simulink model "simgoid_terry"  (R2020b)
settings: Solver=VariableStepAuto  StartTime=0.0  StopTime=200  RelTol=1e-3
values from neighbouring files (symbols this model uses):
  A_2 = zeros(3)    [Trial_Script.m]
  B_2 = I_inv    [Trial_Script.m]
  C_2 = eye(3)    [Trial_Script.m]
  D_2 = zeros(3)    [Trial_Script.m]
libraries: mpclib x1, fuzblock x1, cstblocks x1
settings Model: Creator=Jonathan van Zyl  LastModifiedBy=Jonathan van Zyl

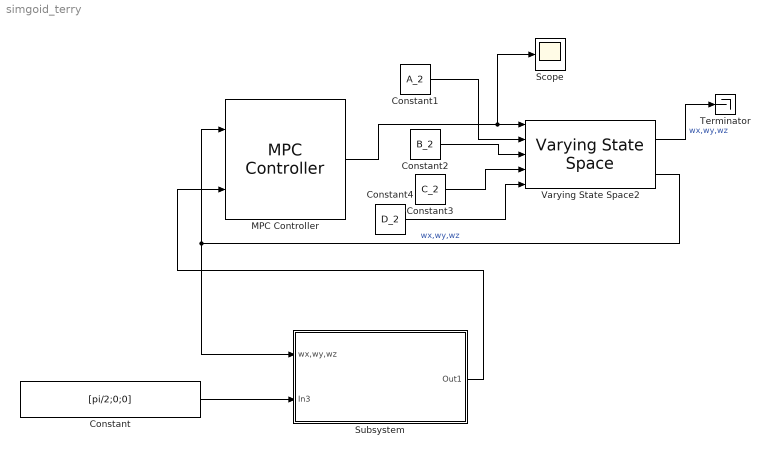
== system simgoid_terry ==
  Constant : Constant  Value=[pi/2;0;0]
  Constant1 : Constant  Value=A_2
  Constant2 : Constant  Value=B_2
  Constant3 : Constant  Value=C_2
  Constant4 : Constant  Value=D_2
  MPC Controller : mpclib/MPC Controller  SCDEnableBlockLinearizationSpecification=on  mpcobj=mpc1  is_multiple=0  enable_value=0  return_u0=off  updateMPCinCallerWorkspace=on  md_inport=off  mv_inport=off  uref_inport=off  return_cost=off  return_mvseq=off  return_qpstatus=off  return_xseq=off  return_state=off  return_ovseq=off  state_inport=off  umin_inport=off  umax_inport=off  ymin_inport=off  ymax_inport=off  cc_inport=off  ywt_inport=off  uwt_inport=off  duwt_inport=off  rhoeps_inport=off  pm_inport=off  MaximumP=10  HorizonChoice=FixedHorizon  n_ts=0.1  n_p=10  n_mv=3  n_md=0  n_ud=0  n_mo=3  n_uo=0  BlockDataType=double  SampleTimeInherited=off  switch_inport=off
  Scope : Scope
  Subsystem : Subsystem
  Terminator : Terminator
  Varying State Space2 : cstblocks/Linear Parameter Varying/Varying State Space  x0=0  xNames=''  OutputX=on  OutputDX=off
  wires:
  Constant3/1 -> Varying State Space2/4
  MPC Controller/1 -> Varying State Space2/1, Scope/1
  Constant2/1 -> Varying State Space2/3
  Varying State Space2/1 -> Terminator/1  "wx,wy,wz"
  Constant4/1 -> Varying State Space2/5
  Varying State Space2/2 -> MPC Controller/1, Subsystem/1(wx,wy,wz)  "wx,wy,wz"
  Constant1/1 -> Varying State Space2/2
  Constant/1 -> Subsystem/2(In3)
  Subsystem/1(Out1) -> MPC Controller/2

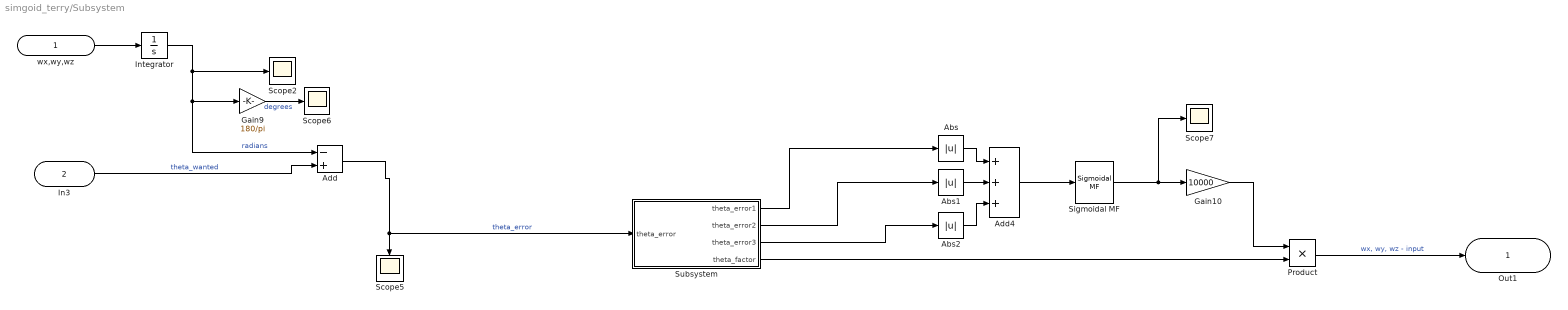
== system simgoid_terry/Subsystem ==
  wx,wy,wz : Inport
  In3 : Inport  Port=2
  Abs : Abs
  Abs1 : Abs
  Abs2 : Abs
  Add : Sum  Inputs=-+
  Add4 : Sum  Inputs=+++
  Gain10 : Gain  Gain=10000
  Gain9 : Gain  Gain=180/pi
  Integrator : Integrator
  Product : Product
  Scope{2,5..7} (4 alike) : Scope
  Sigmoidal MF : fuzblock/Membership  Functions/Sigmoidal MF  a=2.5  c=1.75
      settings: SourceProductBaseCode=FL
  Subsystem : Subsystem
  Out1 : Outport
  wires:
  Integrator/1 -> Add/1, Gain9/1, Scope2/1  "radians"
  Add/1 -> Subsystem/1(theta_error), Scope5/1  "theta_error"
  Abs2/1 -> Add4/3
  Abs1/1 -> Add4/2
  Gain9/1 -> Scope6/1  "degrees"
  Abs/1 -> Add4/1
  Gain10/1 -> Product/1
  Sigmoidal MF/1 -> Scope7/1, Gain10/1
  Add4/1 -> Sigmoidal MF/1
  In3/1 -> Add/2  "theta_wanted"
  Product/1 -> Out1/1  "wx, wy, wz - input"
  wx,wy,wz/1 -> Integrator/1
  Subsystem/1(theta_error1) -> Abs/1
  Subsystem/2(theta_error2) -> Abs1/1
  Subsystem/3(theta_error3) -> Abs2/1
  Subsystem/4(theta_factor) -> Product/2

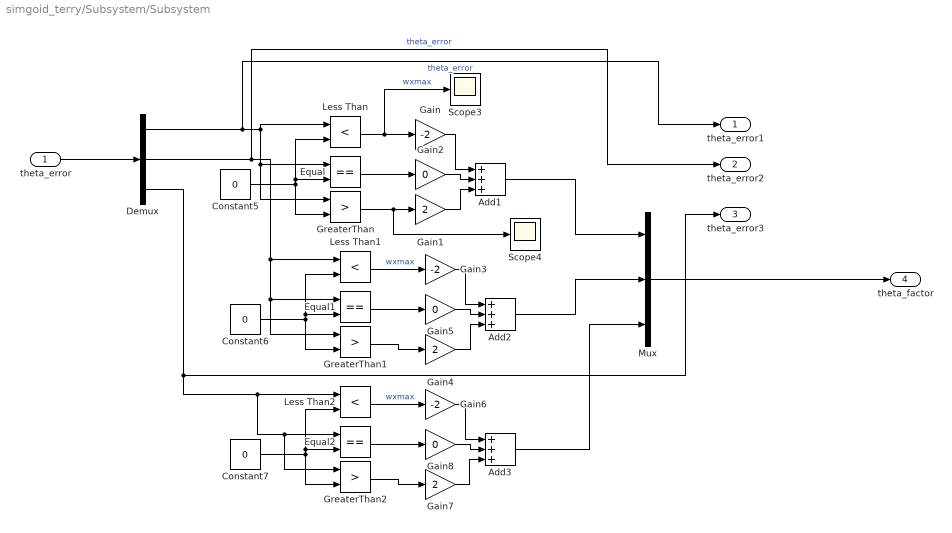
== system simgoid_terry/Subsystem/Subsystem ==
  theta_error : Inport
  Add1 : Sum  Inputs=+++
  Add2 : Sum  Inputs=+++
  Add3 : Sum  Inputs=+++
  Constant5 : Constant  Value=0
  Constant6 : Constant  Value=0
  Constant7 : Constant  Value=0
  Demux : Demux  Outputs=3
  Equal : RelationalOperator  Operator===  OutDataTypeStr=boolean  RndMeth=Simplest
  Equal1 : RelationalOperator  Operator===  OutDataTypeStr=boolean  RndMeth=Simplest
  Equal2 : RelationalOperator  Operator===  OutDataTypeStr=boolean  RndMeth=Simplest
  Gain : Gain  Gain=-2
  Gain1 : Gain  Gain=2
  Gain2 : Gain  Gain=0
  Gain3 : Gain  Gain=-2
  Gain4 : Gain  Gain=2
  Gain5 : Gain  Gain=0
  Gain6 : Gain  Gain=-2
  Gain7 : Gain  Gain=2
  Gain8 : Gain  Gain=0
  GreaterThan : RelationalOperator  Operator=>  OutDataTypeStr=boolean  RndMeth=Simplest
  GreaterThan1 : RelationalOperator  Operator=>  OutDataTypeStr=boolean  RndMeth=Simplest
  GreaterThan2 : RelationalOperator  Operator=>  OutDataTypeStr=boolean  RndMeth=Simplest
  Less Than : RelationalOperator  Operator=<  OutDataTypeStr=boolean  RndMeth=Simplest
  Less Than1 : RelationalOperator  Operator=<  OutDataTypeStr=boolean  RndMeth=Simplest
  Less Than2 : RelationalOperator  Operator=<  OutDataTypeStr=boolean  RndMeth=Simplest
  Mux : Mux  Inputs=3
  Scope3 : Scope
  Scope4 : Scope
  theta_error1 : Outport
  theta_error2 : Outport  Port=2
  theta_error3 : Outport  Port=3
  theta_factor : Outport  Port=4
  wires:
  Add1/1 -> Mux/1
  Constant5/1 -> Equal/2, Less Than/2, GreaterThan/2
  Equal2/1 -> Gain8/1
  Demux/1 -> theta_error1/1, GreaterThan/1, Equal/1, Less Than/1  "theta_error"
  GreaterThan2/1 -> Gain7/1
  Gain1/1 -> Add1/3
  Gain7/1 -> Add3/3
  Less Than1/1 -> Gain3/1  "wxmax"
  Gain6/1 -> Add3/1
  Equal/1 -> Gain2/1
  Gain5/1 -> Add2/2
  Add3/1 -> Mux/3
  GreaterThan/1 -> Scope4/1, Gain1/1
  Constant6/1 -> Equal1/2, Less Than1/2, GreaterThan1/2
  Demux/3 -> theta_error3/1, GreaterThan2/1, Equal2/1, Less Than2/1
  Gain3/1 -> Add2/1
  Constant7/1 -> Equal2/2, Less Than2/2, GreaterThan2/2
  Equal1/1 -> Gain5/1
  Gain8/1 -> Add3/2
  Gain4/1 -> Add2/3
  GreaterThan1/1 -> Gain4/1
  Gain/1 -> Add1/1
  Demux/2 -> theta_error2/1, GreaterThan1/1, Equal1/1, Less Than1/1  "theta_error"
  Gain2/1 -> Add1/2
  Add2/1 -> Mux/2
  Less Than/1 -> Scope3/1, Gain/1  "wxmax"
  Less Than2/1 -> Gain6/1  "wxmax"
  theta_error/1 -> Demux/1
  Mux/1 -> theta_factor/1
